simulink model "FIVE_BUS"  (R2024b)
settings: Solver=VariableStepAuto  StartTime=0.0  StopTime=10.0  RelTol=1e-3
libraries: spsThreePhaseSeriesRLCBranchLib x12, spsGroundLib x7, spsThreePhaseVIMeasurementLib x5, spsLoadFlowBusLib x5, spsThreePhaseSeriesRLCLoadLib x4, spsThreePhaseProgrammableVoltageSourceLib x2, sps_lib x1
settings Model: Creator=Liliane  LastModifiedBy=SamuelCanario

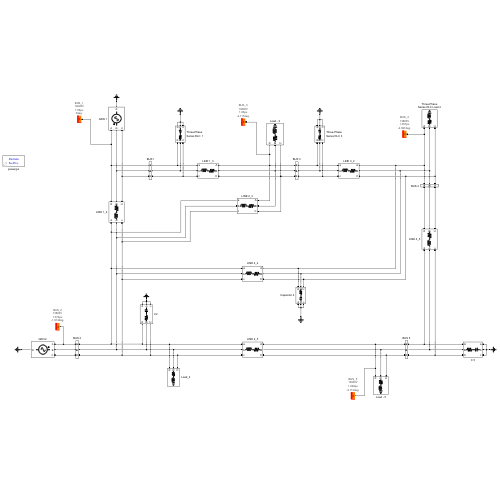
[thumbnail: Simulink's stored preview of the top-level diagram]
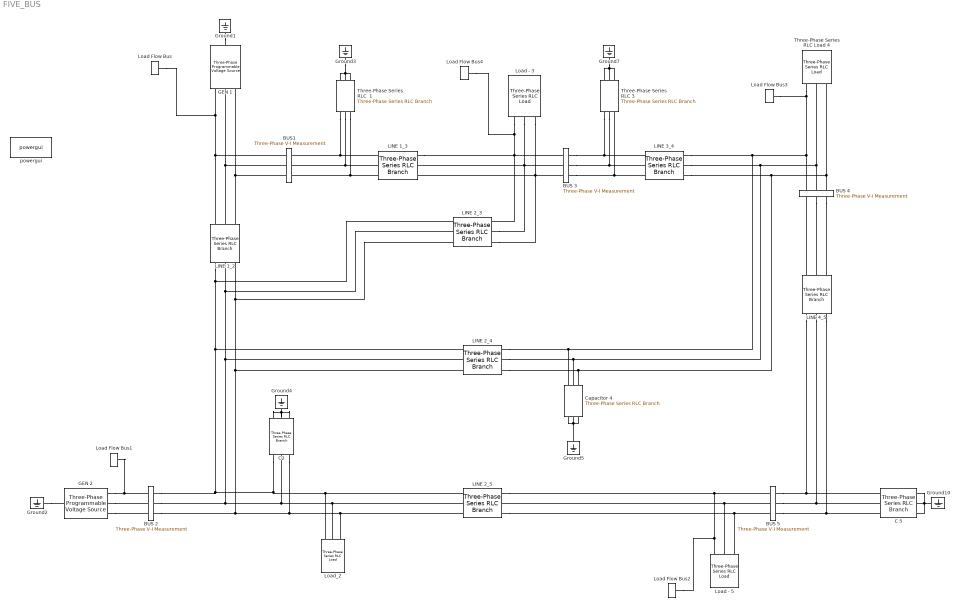
== system FIVE_BUS ==
  " Load - 5" : spsThreePhaseSeriesRLCLoadLib/Three-Phase Series RLC Load  LConnTagsString=A|B|C  Configuration=Y (grounded)  NominalVoltage=(15000)*1.04778  Vabc=[1e3 1e3 1e3]  Vabcp=[1e3 1e3 1e3]  NominalFrequency=60  UnbalancedPower=off  ActivePower=60000000  InductivePower=10000000  CapacitivePower=0  Pabc=[10e3 9e3 11e3]  QLabc=[100 90 110]  QCabc=[100 90 110]  Pabcp=[10e3 9e3 11e3]  QLabcp=[100 90 110]  QCabcp=[100 90 110]  Measurements=None  LoadType=constant PQ
  BUS {2..5} (4 alike) : spsThreePhaseVIMeasurementLib/Three-Phase V-I Measurement  VoltageMeasurement=no  SetLabelV=off  LabelV=Vabc  Vpu=off  VpuLL=off  CurrentMeasurement=no  SetLabelI=off  LabelI=Iabc  Ipu=off  Pbase=100e6  Vbase=500e3  OutputType=Complex  PhasorSimulation=off  PSBequivalent=0
  BUS1 : spsThreePhaseVIMeasurementLib/Three-Phase V-I Measurement  VoltageMeasurement=no  SetLabelV=off  LabelV=Vabc  Vpu=off  VpuLL=off  CurrentMeasurement=no  SetLabelI=off  LabelI=Iabc  Ipu=off  Pbase=100e6  Vbase=500e3  OutputType=Complex  PhasorSimulation=off  PSBequivalent=0
  C 5 : spsThreePhaseSeriesRLCBranchLib/Three-Phase Series RLC Branch  LConnTagsString=A|B|C  RConnTagsString=A|B|C  BranchType=RC  Resistance=0.0001  Inductance=1e-3  Capacitance=5.57E-05  Measurements=None
  C2 : spsThreePhaseSeriesRLCBranchLib/Three-Phase Series RLC Branch  LConnTagsString=A|B|C  RConnTagsString=A|B|C  BranchType=RC  Resistance=0.0001  Inductance=1e-3  Capacitance=0.000118  Measurements=None
  Capacitor 4 : spsThreePhaseSeriesRLCBranchLib/Three-Phase Series RLC Branch  LConnTagsString=A|B|C  RConnTagsString=A|B|C  BranchType=RC  Resistance=0.0001  Inductance=1e-3  Capacitance=7.66e-5  Measurements=None
  GEN 1 : spsThreePhaseProgrammableVoltageSourceLib/Three-Phase Programmable Voltage Source  PositiveSequence=[(14628) 0 60]  VariationEntity=None  VariationType=Table of time-amplitude pairs  VariationTypeAlt=Step  VariationStep=0.5  VariationRate=10  VariationMagnitude=0.3  VariationFrequency=2  VariationTiming=[1 2]  VariationPhaseA=off  Amplitudes=[1 0.8 1.2 1.0]  TimeValues=[0 0.1 0.15 0.2]  HarmonicGeneration=off  HarmonicA=[3 0.2 -25 0]  HarmonicB=[2 0.15 35 2]  Timing="[0.05  3]"  BusType=swing  Pref=40E6  Qref=0  Qmin=-Inf  Qmax=Inf
  GEN 2 : spsThreePhaseProgrammableVoltageSourceLib/Three-Phase Programmable Voltage Source  PositiveSequence=[13.8e3 0 60]  VariationEntity=None  VariationType=Table of time-amplitude pairs  VariationTypeAlt=Step  VariationStep=0.5  VariationRate=10  VariationMagnitude=0.3  VariationFrequency=2  VariationTiming=[1 2]  VariationPhaseA=off  Amplitudes=[1 0.8 1.2 1.0]  TimeValues=[0 0.1 0.15 0.2]  HarmonicGeneration=off  HarmonicA=[3 0.2 -25 0]  HarmonicB=[2 0.15 35 2]  Timing="[0.05  3]"  BusType=PQ  Pref=40000000  Qref=30000000  Qmin=0  Qmax=0
  Ground{1..5,7,10} (7 alike) : spsGroundLib/Ground  LConnTagsString=a
  LINE 1_2 : spsThreePhaseSeriesRLCBranchLib/Three-Phase Series RLC Branch  LConnTagsString=A|B|C  RConnTagsString=A|B|C  BranchType=RL  Resistance=0.0381  Inductance=0.000303  Capacitance=1e-6  Measurements=None
  LINE 1_3 : spsThreePhaseSeriesRLCBranchLib/Three-Phase Series RLC Branch  LConnTagsString=A|B|C  RConnTagsString=A|B|C  BranchType=RL  Resistance=0.152352  Inductance=0.001212  Capacitance=1e-6  Measurements=None
  LINE 2_3 : spsThreePhaseSeriesRLCBranchLib/Three-Phase Series RLC Branch  LConnTagsString=A|B|C  RConnTagsString=A|B|C  BranchType=RL  Resistance=0.114264  Inductance=0.000909  Capacitance=1e-6  Measurements=None
  LINE 2_4 : spsThreePhaseSeriesRLCBranchLib/Three-Phase Series RLC Branch  LConnTagsString=A|B|C  RConnTagsString=A|B|C  BranchType=RL  Resistance=0.114264  Inductance=0.000909  Capacitance=1e-6  Measurements=None
  LINE 2_5 : spsThreePhaseSeriesRLCBranchLib/Three-Phase Series RLC Branch  LConnTagsString=A|B|C  RConnTagsString=A|B|C  BranchType=RL  Resistance=0.076176  Inductance=0.000606  Capacitance=1e-6  Measurements=None
  LINE 3_4 : spsThreePhaseSeriesRLCBranchLib/Three-Phase Series RLC Branch  LConnTagsString=A|B|C  RConnTagsString=A|B|C  BranchType=RL  Resistance=0.019044  Inductance=0.000152  Capacitance=1e-6  Measurements=None
  LINE 4_5 : spsThreePhaseSeriesRLCBranchLib/Three-Phase Series RLC Branch  LConnTagsString=A|B|C  RConnTagsString=A|B|C  BranchType=RL  Resistance=0.152352  Inductance=0.001212  Capacitance=1e-6  Measurements=None
  Load - 3 : spsThreePhaseSeriesRLCLoadLib/Three-Phase Series RLC Load  LConnTagsString=A|B|C  Configuration=Y (grounded)  NominalVoltage=(15000)*1.06033  Vabc=[1e3 1e3 1e3]  Vabcp=[1e3 1e3 1e3]  NominalFrequency=60  UnbalancedPower=off  ActivePower=45000000  InductivePower=15000000  CapacitivePower=0  Pabc=[10e3 9e3 11e3]  QLabc=[100 90 110]  QCabc=[100 90 110]  Pabcp=[10e3 9e3 11e3]  QLabcp=[100 90 110]  QCabcp=[100 90 110]  Measurements=None  LoadType=constant PQ
  Load Flow Bus : spsLoadFlowBusLib/Load Flow Bus  LConnTagsString=a  Phases=single  Connectors=on one side  ID=BUS_1  Vbase=14628  Vref=1  Vangle=0  VLF=1.06  VLFb=1  VLFc=1  angleLF=0  angleLFb=0  angleLFc=0
  Load Flow Bus1 : spsLoadFlowBusLib/Load Flow Bus  LConnTagsString=a  Phases=single  Connectors=on one side  ID=BUS_2  Vbase=13800  Vref=1  Vangle=0  VLF=1.074  VLFb=1  VLFc=1  angleLF=-1.914  angleLFb=0  angleLFc=0
  Load Flow Bus2 : spsLoadFlowBusLib/Load Flow Bus  LConnTagsString=a  Phases=single  Connectors=on one side  ID=BUS_5  Vbase=13800  Vref=1  Vangle=0  VLF=1.048  VLFb=1  VLFc=1  angleLF=-5.112  angleLFb=0  angleLFc=0
  Load Flow Bus3 : spsLoadFlowBusLib/Load Flow Bus  LConnTagsString=a  Phases=single  Connectors=on one side  ID=BUS_4  Vbase=13800  Vref=1  Vangle=0  VLF=1.057  VLFb=1  VLFc=1  angleLF=-4.391  angleLFb=0  angleLFc=0
  Load Flow Bus4 : spsLoadFlowBusLib/Load Flow Bus  LConnTagsString=a  Phases=single  Connectors=on one side  ID=BUS_3  Vbase=13800  Vref=1  Vangle=0  VLF=1.06  VLFb=1  VLFc=1  angleLF=-4.117  angleLFb=0  angleLFc=0
  Load_2 : spsThreePhaseSeriesRLCLoadLib/Three-Phase Series RLC Load  LConnTagsString=A|B|C  Configuration=Y (grounded)  NominalVoltage=(15000)*1.07402  Vabc=[1e3 1e3 1e3]  Vabcp=[1e3 1e3 1e3]  NominalFrequency=60  UnbalancedPower=off  ActivePower=20000000  InductivePower=10000000  CapacitivePower=0  Pabc=[10e3 9e3 11e3]  QLabc=[100 90 110]  QCabc=[100 90 110]  Pabcp=[10e3 9e3 11e3]  QLabcp=[100 90 110]  QCabcp=[100 90 110]  Measurements=None  LoadType=constant PQ
  Three-Phase Series RLC  1 : spsThreePhaseSeriesRLCBranchLib/Three-Phase Series RLC Branch  LConnTagsString=A|B|C  RConnTagsString=A|B|C  BranchType=RC  Resistance=0.0001  Inductance=1e-3  Capacitance=(6.488e-5)  Measurements=None
  Three-Phase Series RLC 3 : spsThreePhaseSeriesRLCBranchLib/Three-Phase Series RLC Branch  LConnTagsString=A|B|C  RConnTagsString=A|B|C  BranchType=RC  Resistance=0.0001  Inductance=1e-3  Capacitance=(7.66e-5)  Measurements=None
  Three-Phase Series RLC Load 4 : spsThreePhaseSeriesRLCLoadLib/Three-Phase Series RLC Load  LConnTagsString=A|B|C  Configuration=Y (grounded)  NominalVoltage=(15000)*1.05738  Vabc=[1e3 1e3 1e3]  Vabcp=[1e3 1e3 1e3]  NominalFrequency=60  UnbalancedPower=off  ActivePower=40000000  InductivePower=5000000  CapacitivePower=0  Pabc=[10e3 9e3 11e3]  QLabc=[100 90 110]  QCabc=[100 90 110]  Pabcp=[10e3 9e3 11e3]  QLabcp=[100 90 110]  QCabcp=[100 90 110]  Measurements=None  LoadType=constant PQ
  powergui : sps_lib/powergui  Priority=1  SimulationMode=Discrete  SampleTime=50e-6  frequency=60  Iterations=50  frequencyindice=60  Pbase=100e6  ErrMax=1e-4  UnitsV=kV  UnitsW=MW  buscounter=0  FunctionMessages=off  echomessages=off  EnableUseOfTLC=off  CurrentSourceSwitches=off  DisableSnubberDevices=off  DisableRonSwitches=off  DisableVfSwitches=off  DisplayEquations=off  AutomaticDiscreteSolvers=off  SolverType=Tustin/Backward Euler (TBE)  Interpol=off  ExternalGateDelay=off  methode=off  Ts=100  x0status=blocks  SPID=on  SwTol=0  HookPort=off  NonlinearTolerance=1e-4  nMaxIteration=100  ContinueOnMaxIteration=off  RestoreLinks=warning  ResistiveCurrentMeasurement=off  Frange=[0:2:500]  Ylog=off  Xlog=on  ShowGrid=off  save=off  variable=ZData  structure=0  ZoomFFT=off  StartTime=0.0  cycles=1  DisplayStyle=1  fundamental=60  FreqAxis=off  MaxFrequency=1000  frequencyindicesteady=1  RmsSteady=1  display=off
  connections:
  Load Flow Bus/LConn1 -- BUS1/RConn1 -- LINE 1_2/LConn1 -- GEN 1/RConn1
  Three-Phase Series RLC  1/LConn1 -- BUS1/LConn1 -- LINE 1_3/RConn1
  LINE 2_4/RConn1 -- BUS 2/LConn1 -- LINE 2_5/RConn1 -- Load_2/LConn1 -- C2/LConn1 -- LINE 2_3/RConn1 -- LINE 1_2/RConn1
  Load_2/LConn3 -- LINE 2_5/RConn3 -- C2/LConn3 -- BUS 2/LConn3 -- LINE 2_3/RConn3 -- LINE 1_2/RConn3 -- LINE 2_4/RConn3
  Three-Phase Series RLC  1/RConn2 -- Ground3/LConn1 -- Three-Phase Series RLC  1/RConn1 -- Three-Phase Series RLC  1/RConn3
  BUS 4/RConn3 -- LINE 4_5/LConn3
  BUS 4/RConn2 -- LINE 4_5/LConn2
  Ground7/LConn1 -- Three-Phase Series RLC 3/RConn2 -- Three-Phase Series RLC 3/RConn3 -- Three-Phase Series RLC 3/RConn1
  LINE 4_5/RConn3 -- BUS 5/LConn3 -- C 5/LConn3
  LINE 4_5/RConn2 -- BUS 5/LConn2 -- C 5/LConn2
  LINE 4_5/RConn1 -- BUS 5/LConn1 -- C 5/LConn1
  LINE 3_4/LConn1 -- LINE 2_4/LConn1 -- Capacitor 4/LConn1 -- Load Flow Bus3/LConn1 -- Three-Phase Series RLC Load 4/LConn1 -- BUS 4/LConn1
  LINE 2_4/LConn2 -- BUS 4/LConn2 -- Three-Phase Series RLC Load 4/LConn2 -- LINE 3_4/LConn2 -- Capacitor 4/LConn2
  LINE 2_4/LConn3 -- BUS 4/LConn3 -- Three-Phase Series RLC Load 4/LConn3 -- LINE 3_4/LConn3 -- Capacitor 4/LConn3
  LINE 2_3/LConn3 -- Load - 3/LConn3 -- LINE 1_3/LConn3 -- BUS 3/RConn3
  LINE 2_3/LConn2 -- LINE 1_3/LConn2 -- Load - 3/LConn2 -- BUS 3/RConn2
  LINE 1_3/LConn1 -- Load Flow Bus4/LConn1 -- Load - 3/LConn1 -- BUS 3/RConn1 -- LINE 2_3/LConn1
  C 5/RConn3 -- C 5/RConn1 -- Ground10/LConn1 -- C 5/RConn2
  Three-Phase Series RLC  1/LConn2 -- BUS1/LConn2 -- LINE 1_3/RConn2
  Three-Phase Series RLC  1/LConn3 -- BUS1/LConn3 -- LINE 1_3/RConn3
  LINE 1_2/LConn3 -- GEN 1/RConn3 -- BUS1/RConn3
  LINE 1_2/LConn2 -- BUS1/RConn2 -- GEN 1/RConn2
  LINE 3_4/RConn3 -- BUS 3/LConn3 -- Three-Phase Series RLC 3/LConn3
  Three-Phase Series RLC 3/LConn2 -- BUS 3/LConn2 -- LINE 3_4/RConn2
  Three-Phase Series RLC 3/LConn1 -- BUS 3/LConn1 -- LINE 3_4/RConn1
  LINE 4_5/LConn1 -- BUS 4/RConn1
  LINE 2_5/LConn3 -- " Load - 5"/LConn3 -- BUS 5/RConn3
  BUS 5/RConn2 -- LINE 2_5/LConn2 -- " Load - 5"/LConn2
  LINE 2_5/LConn1 -- Load Flow Bus2/LConn1 -- " Load - 5"/LConn1 -- BUS 5/RConn1
  Ground2/LConn1 -- GEN 2/LConn1
  LINE 2_5/RConn2 -- Load_2/LConn2 -- BUS 2/LConn2 -- LINE 2_3/RConn2 -- LINE 1_2/RConn2 -- LINE 2_4/RConn2 -- C2/LConn2
  C2/RConn1 -- C2/RConn3 -- Ground4/LConn1 -- C2/RConn2
  Ground1/LConn1 -- GEN 1/LConn1
  Ground5/LConn1 -- Capacitor 4/RConn3 -- Capacitor 4/RConn1 -- Capacitor 4/RConn2
  GEN 2/RConn2 -- BUS 2/RConn2
  GEN 2/RConn3 -- BUS 2/RConn3
  GEN 2/RConn1 -- Load Flow Bus1/LConn1 -- BUS 2/RConn1
